simulink model "ECE_431_Homework_2"  (R2017a)
settings: Solver=VariableStepAuto  StartTime=0.0  StopTime=10.0  RelTol=1e-3
libraries: powerlib x10
settings Model: Creator=Kenzie Brian  LastModifiedBy=Kenzie Brian

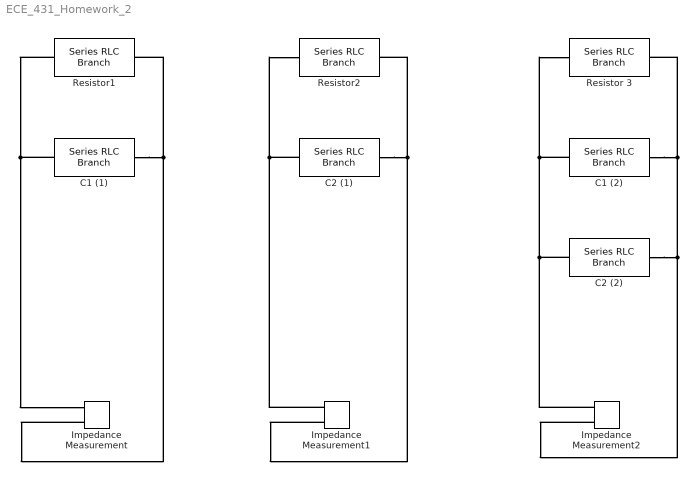
== system ECE_431_Homework_2 ==
  C1 (1) : powerlib/Elements/Series RLC Branch  LConnTagsString=__new0  RConnTagsString=__new0  BranchType=RLC  Resistance=.037  Inductance=16e-9  SetiL0=off  InitialCurrent=0  Capacitance=680e-6  Setx0=off  InitialVoltage=0  Measurements=None
  C1 (2) : powerlib/Elements/Series RLC Branch  LConnTagsString=__new0  RConnTagsString=__new0  BranchType=RLC  Resistance=.037  Inductance=16e-9  SetiL0=off  InitialCurrent=0  Capacitance=680e-6  Setx0=off  InitialVoltage=0  Measurements=None
  C2 (1) : powerlib/Elements/Series RLC Branch  LConnTagsString=__new0  RConnTagsString=__new0  BranchType=RLC  Resistance=.04  Inductance=34e-9  SetiL0=off  InitialCurrent=0  Capacitance=10e-6  Setx0=off  InitialVoltage=0  Measurements=None
  C2 (2) : powerlib/Elements/Series RLC Branch  LConnTagsString=__new0  RConnTagsString=__new0  BranchType=RLC  Resistance=.04  Inductance=34e-9  SetiL0=off  InitialCurrent=0  Capacitance=10e-6  Setx0=off  InitialVoltage=0  Measurements=None
  Impedance Measurement : powerlib/Measurements/Impedance Measurement  LConnTagsString=+|-  Factor=1
      settings: SourceProductName=Simscape Power Systems  SourceProductBaseCode=PS
  Impedance Measurement1 : powerlib/Measurements/Impedance Measurement  LConnTagsString=+|-  Factor=1
      settings: SourceProductName=Simscape Power Systems  SourceProductBaseCode=PS
  Impedance Measurement2 : powerlib/Measurements/Impedance Measurement  LConnTagsString=+|-  Factor=1
      settings: SourceProductName=Simscape Power Systems  SourceProductBaseCode=PS
  Resistor 3 : powerlib/Elements/Series RLC Branch  LConnTagsString=__new0  RConnTagsString=__new0  BranchType=RLC  Resistance=1e12  Inductance=0  SetiL0=off  InitialCurrent=0  Capacitance=0  Setx0=off  InitialVoltage=0  Measurements=None
  Resistor1 : powerlib/Elements/Series RLC Branch  LConnTagsString=__new0  RConnTagsString=__new0  BranchType=RLC  Resistance=1e12  Inductance=0  SetiL0=off  InitialCurrent=0  Capacitance=0  Setx0=off  InitialVoltage=0  Measurements=None
  Resistor2 : powerlib/Elements/Series RLC Branch  LConnTagsString=__new0  RConnTagsString=__new0  BranchType=RLC  Resistance=1e12  Inductance=0  SetiL0=off  InitialCurrent=0  Capacitance=0  Setx0=off  InitialVoltage=0  Measurements=None
  connections:
  Resistor1/LConn1 -- C1 (1)/LConn1 -- Impedance Measurement/LConn1
  Impedance Measurement/LConn2 -- C1 (1)/RConn1 -- Resistor1/RConn1
  Impedance Measurement1/LConn1 -- C2 (1)/LConn1 -- Resistor2/LConn1
  Impedance Measurement1/LConn2 -- C2 (1)/RConn1 -- Resistor2/RConn1
  Impedance Measurement2/LConn1 -- C2 (2)/LConn1 -- C1 (2)/LConn1 -- Resistor 3/LConn1
  Impedance Measurement2/LConn2 -- C2 (2)/RConn1 -- C1 (2)/RConn1 -- Resistor 3/RConn1
